simulink model "Closed_Loop_System_7D"  (R2019b)
settings: Solver=VariableStepAuto  StartTime=0.0  StopTime=30  RelTol=1e-9
undefined symbols (not defined in the file): A, B, C, eta, F, g, G, H, K, L, m, mu, r, T_bar, x_des
settings Model: Creator=Orkun  LastModifiedBy=ant-x
settings DebuggingCC: UnconnectedInputMsg=none  UnconnectedOutputMsg=none  UnconnectedLineMsg=none  SFMachineParentedDataDiag=error

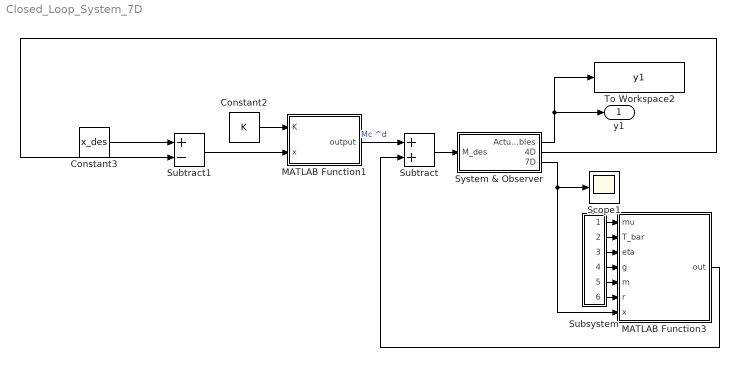
== system Closed_Loop_System_7D ==
  Constant2 : Constant  Value=K  VectorParams1D=off
  Constant3 : Constant  Value=x_des  VectorParams1D=off
  MATLAB Function1 : MATLAB Function  TreatAsAtomicUnit=on
  MATLAB Function3 : MATLAB Function  TreatAsAtomicUnit=on
  Scope1 : Scope
  Subsystem : Subsystem
  Subtract : Sum
  Subtract1 : Sum  Inputs=+-
  System & Observer : Subsystem
  To Workspace2 : ToWorkspace  VariableName=y1  SaveFormat=Timeseries  SampleTime=-1
  y1 : Outport
  wires:
  System & Observer/1(Actual variables) -> To Workspace2/1, y1/1
  MATLAB Function1/1(output) -> Subtract/1  "Mc ^d"
  Constant2/1 -> MATLAB Function1/1(K)
  System & Observer/3(7D) -> MATLAB Function3/7(x), Scope1/1
  System & Observer/2(4D) -> Subtract1/2
  Subtract1/1 -> MATLAB Function1/2(x)
  Subtract/1 -> System & Observer/1(M_des)
  Constant3/1 -> Subtract1/1
  MATLAB Function3/1(out) -> Subtract/2
  Subsystem/1(Out1) -> MATLAB Function3/1(mu)
  Subsystem/2(Out2) -> MATLAB Function3/2(T_bar)
  Subsystem/3(Out3) -> MATLAB Function3/3(eta)
  Subsystem/4(Out4) -> MATLAB Function3/4(g)
  Subsystem/5(Out5) -> MATLAB Function3/5(m)
  Subsystem/6(Out6) -> MATLAB Function3/6(r)

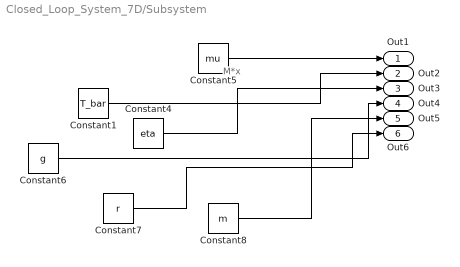
== system Closed_Loop_System_7D/Subsystem ==
  note: M*x
  Constant1 : Constant  Value=T_bar
  Constant4 : Constant  Value=eta
  Constant5 : Constant  Value=mu  VectorParams1D=off
  Constant6 : Constant  Value=g
  Constant7 : Constant  Value=r
  Constant8 : Constant  Value=m
  Out1 : Outport
  Out2 : Outport  Port=2
  Out3 : Outport  Port=3
  Out4 : Outport  Port=4
  Out5 : Outport  Port=5
  Out6 : Outport  Port=6
  wires:
  Constant7/1 -> Out6/1
  Constant8/1 -> Out5/1
  Constant1/1 -> Out2/1
  Constant4/1 -> Out3/1
  Constant5/1 -> Out1/1
  Constant6/1 -> Out4/1

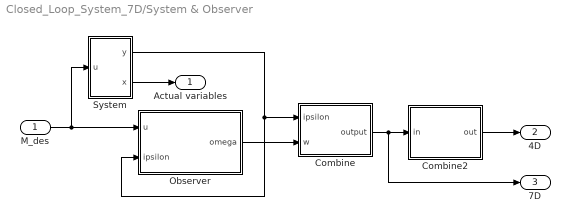
== system Closed_Loop_System_7D/System & Observer ==
  M_des : Inport
  Combine : MATLAB Function  TreatAsAtomicUnit=on
  Combine2 : MATLAB Function  TreatAsAtomicUnit=on
  Observer : Subsystem
  System : Subsystem
  Actual variables : Outport
  4D : Outport  Port=2
  7D : Outport  Port=3
  wires:
  M_des/1 -> System/1(u), Observer/1(u)
  System/1(y) -> Combine/1(ipsilon), Observer/2(ipsilon)
  Observer/1(omega) -> Combine/2(w)
  System/2(x) -> Actual variables/1
  Combine/1(output) -> 7D/1, Combine2/1(in)
  Combine2/1(out) -> 4D/1

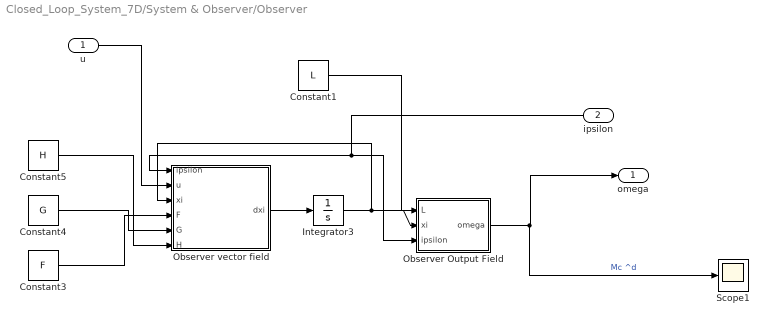
== system Closed_Loop_System_7D/System & Observer/Observer ==
  u : Inport
  ipsilon : Inport  Port=2
  Constant1 : Constant  Value=L  VectorParams1D=off
  Constant3 : Constant  Value=F
  Constant4 : Constant  Value=G
  Constant5 : Constant  Value=H  VectorParams1D=off
  Integrator3 : Integrator  InitialCondition=[0;0;0]
  Observer Output Field : MATLAB Function  TreatAsAtomicUnit=on
  Observer vector field : MATLAB Function  TreatAsAtomicUnit=on
  Scope1 : Scope
  omega : Outport
  wires:
  u/1 -> Observer vector field/2(u)
  Integrator3/1 -> Observer vector field/3(xi), Observer Output Field/2(xi)
  ipsilon/1 -> Observer Output Field/3(ipsilon), Observer vector field/1(ipsilon)
  Constant5/1 -> Observer vector field/6(H)
  Observer vector field/1(dxi) -> Integrator3/1
  Constant4/1 -> Observer vector field/5(G)
  Constant3/1 -> Observer vector field/4(F)
  Observer Output Field/1(omega) -> Scope1/1, omega/1  "Mc ^d"
  Constant1/1 -> Observer Output Field/1(L)

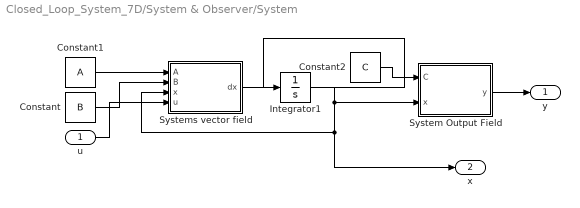
== system Closed_Loop_System_7D/System & Observer/System ==
  u : Inport
  Constant : Constant  Value=B
  Constant1 : Constant  Value=A
  Constant2 : Constant  Value=C
  Integrator1 : Integrator  InitialCondition=[0;0;0;0;0;0;0]
  System Output Field : MATLAB Function  TreatAsAtomicUnit=on
  Systems vector field : MATLAB Function  TreatAsAtomicUnit=on
  y : Outport
  x : Outport  Port=2
  wires:
  Systems vector field/1(dx) -> Integrator1/1
  Constant1/1 -> Systems vector field/1(A)
  Constant2/1 -> System Output Field/1(C)
  u/1 -> Systems vector field/4(u)
  Integrator1/1 -> x/1, Systems vector field/3(x), System Output Field/2(x)
  System Output Field/1(y) -> y/1
  Constant/1 -> Systems vector field/2(B)

== matlab function Closed_Loop_System_7D/System & Observer/Combine2 ==
  data: in input; out output
function out = fcn(in)

out = [in(1,:);in(2,:);in(3,:);in(4,:);];

== matlab function Closed_Loop_System_7D/MATLAB Function3 ==
  data: mu input; T_bar input; eta input; g input; m input; r input; out output; x input
function out = fcn(mu, T_bar, eta, g, m, r, x)
% 
% M = [0,0,0,0;
%     0,0,0,0;
%     0,0,0,0;
%     0,0,0,1]

% intermediate = M*x;
dv = x(6,:);
dq = x(7,:);

% offset = (T_bar*eta*dq + g*m*r*dv )/T_bar*eta*mu;

offset = dq/mu + dv*g*m*r/(T_bar*eta*mu);

out = offset;

== matlab function Closed_Loop_System_7D/MATLAB Function1 ==
  data: K input; output output; x input
function output = fcn(K, x)

output = K*x;

== matlab function Closed_Loop_System_7D/System & Observer/Combine ==
  data: ipsilon input; output output; w input
function output = fcn(ipsilon, w)

output = [ipsilon;w];

== matlab function Closed_Loop_System_7D/System & Observer/Observer/Observer Output Field ==
  data: L input; xi input; omega output; ipsilon input
function omega = fcn(L, xi, ipsilon)

%L = [0, -0.0475; 0, 2.7];

omega = xi + L*ipsilon;

== matlab function Closed_Loop_System_7D/System & Observer/Observer/Observer vector field ==
  data: ipsilon input; u input; dxi output; xi input; F input; G input; H input
function dxi = fcn(ipsilon,u, xi, F, G, H)
%F = [-16.3046, 0.0475; -967.95, -2.7];
%F = [-16.3046, 0; -967.9500, 0];
%G = [33.3333; 0];
%H = [-0.5621, 0.8753; 31.9507, 40.2480];
%H = [-0.5621, 0.747; 31.9507, 47.5382];


dxi = F*xi + H*ipsilon + G*u;

== matlab function Closed_Loop_System_7D/System & Observer/System/System Output Field ==
  data: C input; x input; y output
function y = fcn(C, x)

%C = [1, 0, 0, 0; 0, 1, 0, 0];
y = C*x;

== matlab function Closed_Loop_System_7D/System & Observer/System/Systems vector field ==
  data: A input; B input; x input; u input; dx output
function dx = fcn(A, B, x, u)

dx = (A*x) + (B*u);
